simulink model "Arithemetic_Calculator"  (R2024b)
settings: Solver=VariableStepAuto  StartTime=0.0  StopTime=inf  RelTol=1e-3
settings Model: Creator=rohan  LastModifiedBy=rohan

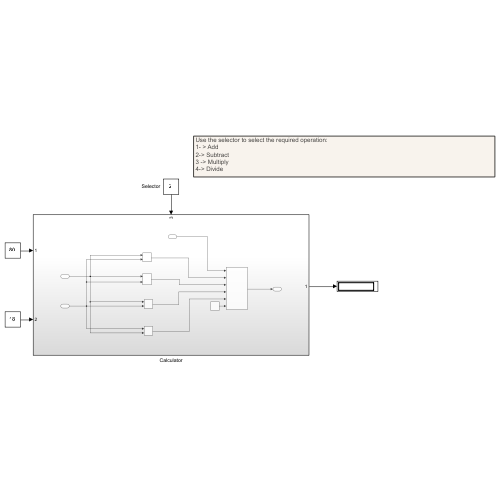
[thumbnail: Simulink's stored preview of the top-level diagram]
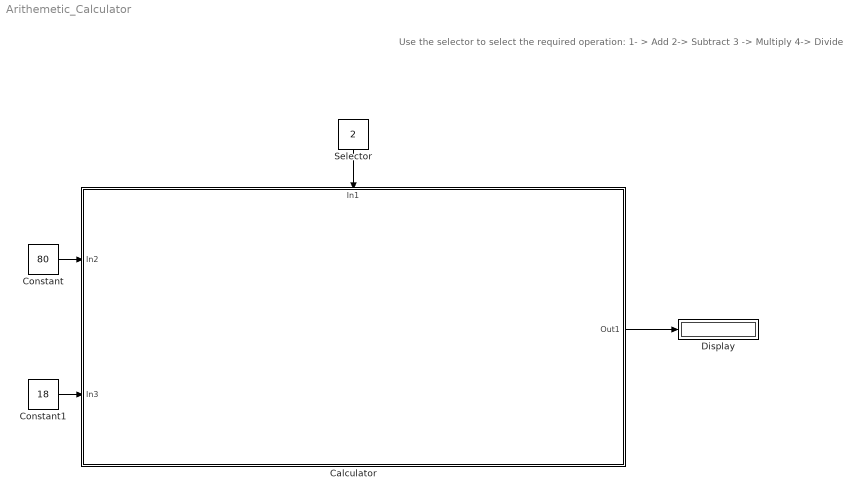
== system Arithemetic_Calculator ==
  note: Use the selector to select the required operation:
      | 1- > Add
      | 2-> Subtract
      | 3 -> Multiply
      | 4-> Divide
  Calculator : Subsystem
      settings: PortSchema="{\"entries\":[{\"content\":{\"sides\":[{\"content\":{\"connectorIds\":[\"In1\",\"In2\"]},\"type\":\"ConnectorPlacement.EquallySpacedRectSide\",\"uuid\":\"b9e9774c-5197-4426-88ea-8c47bb40954b\"},{\"content\":{\"connectorIds\":[\"Out1\"],\"side\":\"RIGHT\"},\"type\":\"ConnectorPlacement.EquallySpacedRectSide\",\"uuid\":\"f25b44e8-8e03-4ae9-b1b4-0ea3e8700d6a\"},{\"content\":{\"connectorIds\":[\"In3\"],\"side\":\"TOP\"},\"type\":\"ConnectorPlacement.EquallySpacedRectSide\",\"uuid\":\"629e52fe-9eb8-4c33-9220-4d58ca333942\"}]},\"type\":\"ConnectorPlacement.EquallySpacedConnector\",\"uuid\":\"b0233f1b-a181-4d6f-a174-cf4610564b50\"}],\"packageUris\":[\"http://schema.mathworks.com/mf0/Connector/R2020b\"],\"version\":\"1.0\"}"
  Constant : Constant  Value=80
  Constant1 : Constant  Value=18
  Display : Display
      settings: Decimation=4
  Selector : Constant  Value=2
  wires:
  Selector/1 -> Calculator/3(In1)
  Constant/1 -> Calculator/1(In2)
  Constant1/1 -> Calculator/2(In3)
  Calculator/1(Out1) -> Display/1

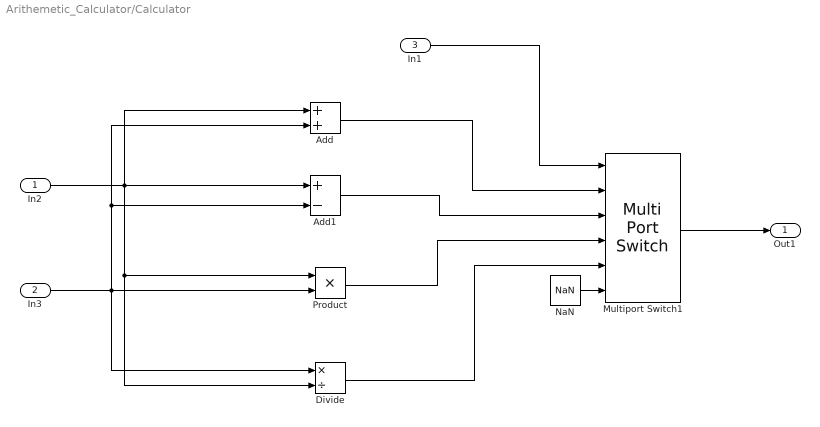
== system Arithemetic_Calculator/Calculator ==
  In2 : Inport
  In3 : Inport  Port=2
  In1 : Inport  Port=3
  Add : Sum
  Add1 : Sum  Inputs=+-
  Divide : Product  Inputs=*/
  Multiport Switch1 : MultiPortSwitch  Inputs=4  DataPortForDefault=Additional data port  DiagnosticForDefault=None  SaturateOnIntegerOverflow=off  InputSameDT=off
  NaN : Constant  Value=NaN  OutDataTypeStr=Inherit: Inherit via back propagation
  Product : Product
  Out1 : Outport
  wires:
  In2/1 -> Add/1, Divide/2, Product/1, Add1/1
  Add1/1 -> Multiport Switch1/3
  NaN/1 -> Multiport Switch1/6
  Product/1 -> Multiport Switch1/4
  In1/1 -> Multiport Switch1/1
  Divide/1 -> Multiport Switch1/5
  In3/1 -> Divide/1, Add/2, Add1/2, Product/2
  Add/1 -> Multiport Switch1/2
  Multiport Switch1/1 -> Out1/1
